simulink model "pendulum_sim"  (R2019b)
settings: Solver=ode45  StartTime=0.0  StopTime=10000  MaxStep=.1  RelTol=1e-3  EnableMultiTasking=on
InitFcn:
  | addpath ./..
  | pendulumParam
undefined symbols (not defined in the file): P, pendulum_animation
libraries: simulink x1
settings Model: Creator=beard  LastModifiedBy=JoHn
settings DataIOCC: LimitDataPoints=on  SaveFormat=Array  SignalLoggingSaveFormat=ModelDataLogs  ReturnWorkspaceOutputs=off
settings OptimizationCC: ExpressionDepthLimit=2147483647  InitFltsAndDblsToZero=on  LifeSpan=inf
settings DebuggingCC: UnderspecifiedInitializationDetection=Classic  MergeDetectMultiDrivingBlocksExec=none  SolverPrmCheckMsg=warning  FcnCallInpInsideContextMsg=warning  StateNameClashWarn=warning  SFUnexpectedBacktrackingDiag=warning  SFNoUnconditionalDefaultTransitionDiag=warning  SFExecutionAtInitializationDiag=none  ArithmeticOperatorsInVariantConditions=warning
settings HardwareCC: ProdBitPerPointer=32  ProdBitPerSizeT=32  ProdBitPerPtrDiffT=32  ProdLargestAtomicFloat=None  ProdIntDivRoundTo=Undefined  ProdEndianess=Unspecified  ProdWordSize=32  ProdHWDeviceType=32-bit Generic
settings ModelReferenceCC: PropagateSignalLabelsOutOfModel=off
settings SFSimCC: SimUseLocalCustomCode=off  CustomCodeUndefinedFunction=UseInterfaceOnly
settings RTWCC: RTWUseLocalCustomCode=off
settings CodeAppCC: StateflowObjectComments=on
settings GRTTargetCC: TargetLangStandard=C89/C90 (ANSI)  GeneratePreprocessorConditionals=Disable all  CombineOutputUpdateFcns=off  GRTInterface=on
settings ConfigComp: CovMetricSettings=dw  CovHtmlReporting=on  CovSaveCumulativeToWorkspaceVar=on  CovSaveSingleToWorkspaceVar=on  CovExternalEMLEnable=off

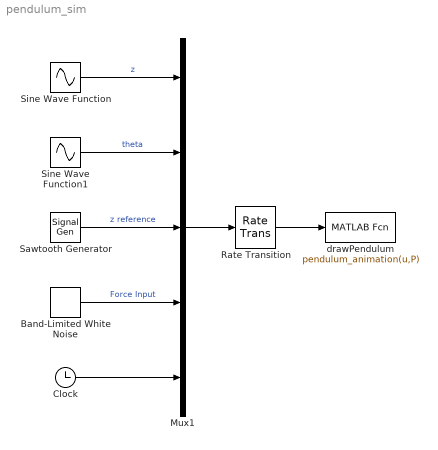
== system pendulum_sim ==
  Band-Limited White Noise : simulink/Sources/Band-Limited White Noise  Cov=[0.1]  Ts=0.1  seed=[23341]
  Clock : Clock
  Mux1 : Mux  Inputs=5
  Rate Transition : RateTransition  OutPortSampleTime=P.t_plot
  Sawtooth Generator : SignalGenerator  WaveForm=sawtooth  Units=rad/sec
  Sine Wave Function : Sin  SampleTime=0
  Sine Wave Function1 : Sin  SampleTime=0
  drawPendulum : MATLABFcn  MATLABFcn=pendulum_animation(u,P)  OutputDimensions=0
  wires:
  Mux1/1 -> Rate Transition/1
  Rate Transition/1 -> drawPendulum/1
  Sine Wave Function/1 -> Mux1/1  "z"
  Sine Wave Function1/1 -> Mux1/2  "theta"
  Sawtooth Generator/1 -> Mux1/3  "z reference"
  Band-Limited White Noise/1 -> Mux1/4  "Force Input"
  Clock/1 -> Mux1/5
